simulink subsystem "Nonlinear_plant"  (R2021b)
settings: Solver=VariableStepAuto  StartTime=0.0  StopTime=10.0  RelTol=1e-3
libraries: simulink x1
settings Model: Creator=aback  LastModifiedBy=aback

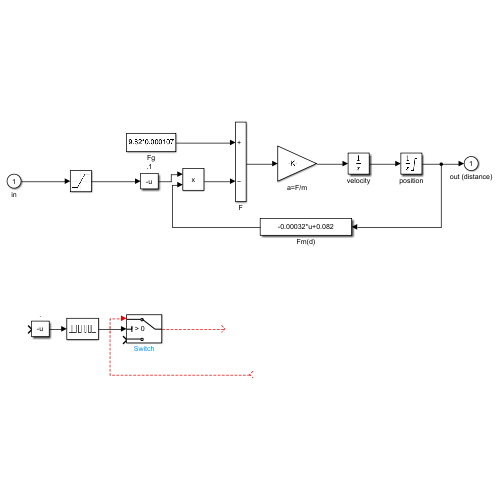
[thumbnail: Simulink's stored preview of the top-level diagram]
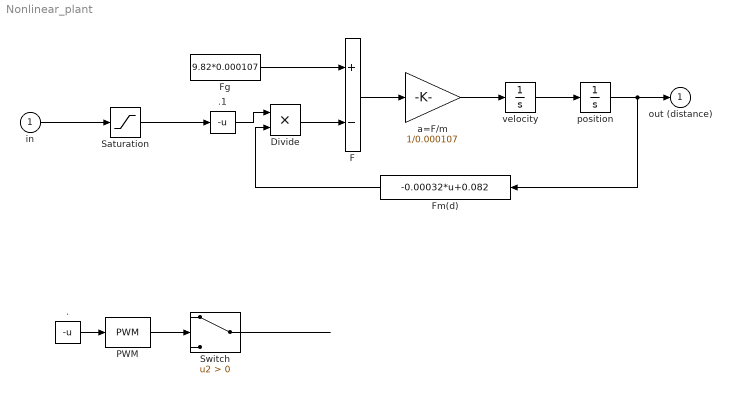
== system Nonlinear_plant ==
  in : Inport
  . : Fcn  StatePerturbationForJacobian=1.0e-05  Expr=-u
  .1 : Fcn  StatePerturbationForJacobian=1.0e-05  Expr=-u
  Divide : Product  Inputs=**
  F : Sum  StatePerturbationForJacobian=1.0e-05  Inputs=+-  InputSameDT=on  SaturateOnIntegerOverflow=on  OutDataTypeStr=Inherit: Same as first input
  Fg : Constant  StatePerturbationForJacobian=1.0e-05  Value=9.82*0.000107  SampleTime=-1
  Fm(d) : Fcn  StatePerturbationForJacobian=1.0e-05  Expr=-0.00032*u+0.082
  PWM : simulink/Discontinuities/PWM  DisableCoverage=on  Period=0.01  DisallowZeroDutyCycle=off  RunAtFixedTimeIntervals=off  SampleTime=0.1
  Saturation : Saturate  UpperLimit=0  LowerLimit=-1
  Switch : Switch  Criteria=u2 > Threshold
  a=F/m : Gain  StatePerturbationForJacobian=1.0e-05  Gain=1/0.000107  SaturateOnIntegerOverflow=on  OutDataTypeStr=Inherit: Same as input  ParamDataTypeStr=Inherit: Same as input
  position : Integrator  StatePerturbationForJacobian=1.0e-05  InitialCondition=15  LimitOutput=on  UpperSaturationLimit=50  LowerSaturationLimit=0  ZeroCross=off
  velocity : Integrator  StatePerturbationForJacobian=1.0e-05  UpperSaturationLimit=1000  LowerSaturationLimit=-1000  ZeroCross=off
  out (distance) : Outport  StatePerturbationForJacobian=1.0e-05
  wires:
  velocity/1 -> position/1
  F/1 -> a=F/m/1
  position/1 -> Fm(d)/1, out (distance)/1
  a=F/m/1 -> velocity/1
  in/1 -> Saturation/1
  Fg/1 -> F/1
  Switch/1 -> ?
  ? -> Switch/1
  PWM/1 -> Switch/2
  ./1 -> PWM/1
  Saturation/1 -> .1/1
  .1/1 -> Divide/1
  Fm(d)/1 -> Divide/2
  Divide/1 -> F/2
